simulink model "TestCellBalance"  (R2022b)
settings: Solver=VariableStepAuto  StartTime=0.0  StopTime=100  RelTol=1e-3
undefined symbols (not defined in the file): Ion, Lithium
libraries: spsSeriesRLCBranchLib x6, spsBatteryLib x4, spsVariableCapacitorLib x4, spsMosfetLib x4, spspowerguiLib x1
settings Model: Creator=49151  LastModifiedBy=49151
settings SolverCC: ZeroCrossAlgorithm=Adaptive
settings DebuggingCC: IgnoredZcDiagnostic=none

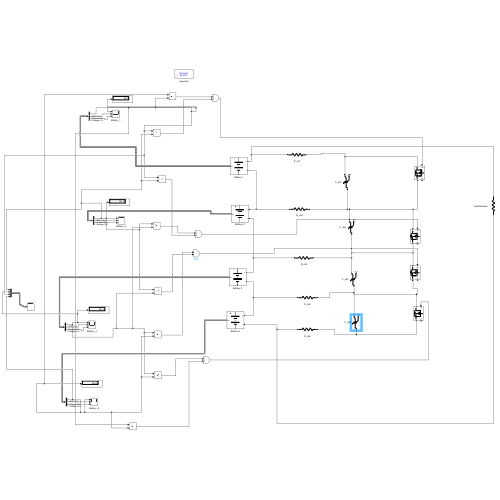
[thumbnail: Simulink's stored preview of the top-level diagram]
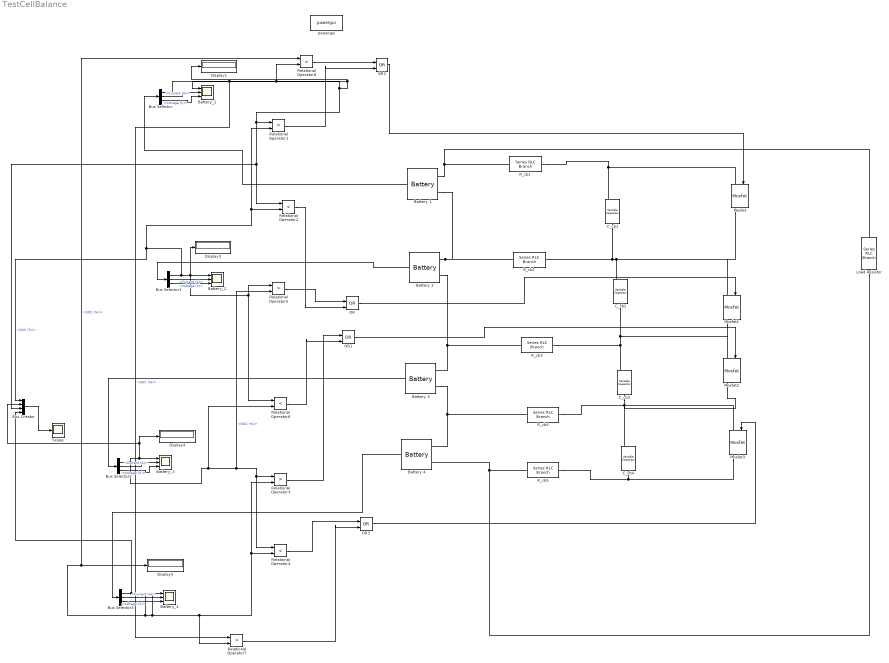
== system TestCellBalance ==
  Battery 1 : spsBatteryLib/Battery  BatType=Lithium-Ion  ShowTempParam=off  ThermalPreset=no  ShowAgeParam=off  NomV=3.7  NomQ=2.6  SOC=97  Batt_Tr=30  PresetModel=on  MaxQ=2.6  MinV=2.775  FullV=4.3068  Dis_rate=1.1304  R=0.014231  Normal_OP=2.3513  expZone="[3.9974     0.12774]"  current=[6.5 13 32.5]  Units=Time  Tci=20  NomT=20  T2=-30  MaxQ2=4.8  FullV2=7.1  Normal_OP2=5.655  expZone2="[6.58           1]"  Rca=0.6  ti=2000  Dp=0  Neq0=0  Tsim=1e6  Ta1=25  Qeol=5.4*0.9  Reol=0.013333*1.2  Char_age=[2.3478, 3]  Dis_age=[2.3478, 10]  N1=1500  N2=10500  N3=1000  N4=1400  Ta2=45  N5=950
  Battery 2 : spsBatteryLib/Battery  BatType=Lithium-Ion  ShowTempParam=off  ThermalPreset=no  ShowAgeParam=off  NomV=3.7  NomQ=2.6  SOC=96  Batt_Tr=30  PresetModel=on  MaxQ=2.6  MinV=2.775  FullV=4.3068  Dis_rate=1.1304  R=0.014231  Normal_OP=2.3513  expZone="[3.9974     0.12774]"  current=[6.5 13 32.5]  Units=Time  Tci=20  NomT=20  T2=-30  MaxQ2=4.8  FullV2=7.1  Normal_OP2=5.655  expZone2="[6.58           1]"  Rca=0.6  ti=2000  Dp=0  Neq0=0  Tsim=1e6  Ta1=25  Qeol=5.4*0.9  Reol=0.013333*1.2  Char_age=[2.3478, 3]  Dis_age=[2.3478, 10]  N1=1500  N2=10500  N3=1000  N4=1400  Ta2=45  N5=950
  Battery 3 : spsBatteryLib/Battery  BatType=Lithium-Ion  ShowTempParam=off  ThermalPreset=no  ShowAgeParam=off  NomV=3.7  NomQ=2.6  SOC=94  Batt_Tr=30  PresetModel=on  MaxQ=2.6  MinV=2.775  FullV=4.3068  Dis_rate=1.1304  R=0.014231  Normal_OP=2.3513  expZone="[3.9974     0.12774]"  current=[6.5 13 32.5]  Units=Time  Tci=20  NomT=20  T2=-30  MaxQ2=4.8  FullV2=7.1  Normal_OP2=5.655  expZone2="[6.58           1]"  Rca=0.6  ti=2000  Dp=0  Neq0=0  Tsim=1e6  Ta1=25  Qeol=5.4*0.9  Reol=0.013333*1.2  Char_age=[2.3478, 3]  Dis_age=[2.3478, 10]  N1=1500  N2=10500  N3=1000  N4=1400  Ta2=45  N5=950
  Battery 4 : spsBatteryLib/Battery  BatType=Lithium-Ion  ShowTempParam=off  ThermalPreset=no  ShowAgeParam=off  NomV=3.7  NomQ=2.6  SOC=96  Batt_Tr=30  PresetModel=on  MaxQ=2.6  MinV=2.775  FullV=4.3068  Dis_rate=1.1304  R=0.014231  Normal_OP=2.3513  expZone="[3.9974     0.12774]"  current=[6.5 13 32.5]  Units=Time  Tci=20  NomT=20  T2=-30  MaxQ2=4.8  FullV2=7.1  Normal_OP2=5.655  expZone2="[6.58           1]"  Rca=0.6  ti=2000  Dp=0  Neq0=0  Tsim=1e6  Ta1=25  Qeol=5.4*0.9  Reol=0.013333*1.2  Char_age=[2.3478, 3]  Dis_age=[2.3478, 10]  N1=1500  N2=10500  N3=1000  N4=1400  Ta2=45  N5=950
  Battery_{1..4} (4 alike) : Scope  NumInputPorts=3
  Bus Creator : BusCreator  Inputs=4
  Bus Selector{,1..3} (4 alike) : BusSelector  OutputSignals=SOC (%),Current (A),Voltage (V)
  C_cb{1..4} (4 alike) : spsVariableCapacitorLib/Variable Capacitor  methode=Backward Euler  Cabsmin=1e-6  Initialize=off  vC0=0  C0=1e-6  iC0=0
      settings: LibrarySourceBlock=sps_lib/Passives/Variable Capacitor
  Display{1,3..5} (4 alike) : Display
  Load Resistor : spsSeriesRLCBranchLib/Series RLC Branch  LConnTagsString=__new0  RConnTagsString=__new0  BranchType=R  Resistance=2  Inductance=1e-3  SetiL0=off  InitialCurrent=0  Capacitance=1e-6  Setx0=off  InitialVoltage=0  Measurements=None
  Mosfet{,1..3} (4 alike) : spsMosfetLib/Mosfet  Ron=0.1  Lon=0  Rd=0.01  Vfd=0  IC=0  Rs=1e5  Cs=inf  Measurements=on
  OR{,1..3} (4 alike) : Logic  Operator=OR  IconShape=distinctive  AllPortsSameDT=off  OutDataTypeStr=boolean
  R_cb{1..5} (5 alike) : spsSeriesRLCBranchLib/Series RLC Branch  LConnTagsString=__new0  RConnTagsString=__new0  BranchType=R  Resistance=1  Inductance=1e-3  SetiL0=off  InitialCurrent=0  Capacitance=1e-6  Setx0=off  InitialVoltage=0  Measurements=None
  Relational Operator{1,3,5,7} (4 alike) : RelationalOperator  Operator=>  OutDataTypeStr=boolean  RndMeth=Simplest  InputSameDT=off
  Relational Operator{2,4,6,8} (4 alike) : RelationalOperator  Operator=<  OutDataTypeStr=boolean  RndMeth=Simplest  InputSameDT=off
  Scope : Scope
  powergui : spspowerguiLib/powergui  Priority=1  SimulationMode=Discrete  SampleTime=50e-6  frequency=60  Iterations=50  frequencyindice=0  Pbase=100e6  ErrMax=1e-4  UnitsV=kV  UnitsW=MW  buscounter=0  FunctionMessages=off  echomessages=off  EnableUseOfTLC=off  CurrentSourceSwitches=off  DisableSnubberDevices=off  DisableRonSwitches=off  DisableVfSwitches=off  DisplayEquations=off  AutomaticDiscreteSolvers=off  SolverType=Tustin/Backward Euler (TBE)  Interpol=off  ExternalGateDelay=off  methode=off  Ts=100  x0status=blocks  SPID=on  SwTol=0  HookPort=off  NonlinearTolerance=1e-4  nMaxIteration=100  ContinueOnMaxIteration=off  RestoreLinks=warning  ResistiveCurrentMeasurement=off  Frange=[0:2:500]  Ylog=off  Xlog=on  ShowGrid=off  save=off  variable=ZData  structure=0  ZoomFFT=off  StartTime=0.0  cycles=1  DisplayStyle=1  fundamental=60  FreqAxis=off  MaxFrequency=1000  frequencyindicesteady=1  RmsSteady=1  display=off
  wires:
  Bus Selector/1 -> Bus Creator/3, Relational Operator2/1, Relational Operator1/1, Display1/1, Relational Operator8/2, Relational Operator7/1, Battery_1/1  "<SOC (%)>"
  Battery 1/1 -> Bus Selector/1
  Bus Selector/3 -> Battery_1/3  "<Voltage (V)>"
  Bus Selector/2 -> Battery_1/2  "<Current (A)>"
  Battery 2/1 -> Bus Selector1/1
  Bus Selector1/1 -> Relational Operator1/2, Relational Operator2/2, Bus Creator/1, Display3/1, Relational Operator5/1, Relational Operator6/1, Battery_2/1  "<SOC (%)>"
  Bus Selector1/2 -> Battery_2/2  "<Current (A)>"
  Bus Selector1/3 -> Battery_2/3  "<Voltage (V)>"
  Relational Operator2/1 -> OR/2
  Bus Selector3/3 -> Battery_4/3  "<Voltage (V)>"
  Bus Selector2/1 -> Battery_3/1, Bus Creator/2, Display4/1, Relational Operator6/2, Relational Operator5/2, Relational Operator4/1, Relational Operator3/1  "<SOC (%)>"
  Bus Selector2/3 -> Battery_3/3  "<Voltage (V)>"
  Battery 4/1 -> Bus Selector3/1
  Bus Selector3/2 -> Battery_4/2  "<Current (A)>"
  Bus Selector2/2 -> Battery_3/2  "<Current (A)>"
  Battery 3/1 -> Bus Selector2/1
  Bus Selector3/1 -> Bus Creator/4, Relational Operator7/2, Relational Operator3/2, Relational Operator4/2, Battery_4/1, Relational Operator8/1, Display5/1  "<SOC (%)>"
  Bus Creator/1 -> Scope/1
  Relational Operator5/1 -> OR/1
  OR/1 -> Mosfet1/1
  OR1/1 -> Mosfet2/1
  Relational Operator3/1 -> OR1/1
  Relational Operator6/1 -> OR1/2
  Relational Operator8/1 -> OR2/1
  Relational Operator1/1 -> OR2/2
  OR2/1 -> Mosfet/1
  Relational Operator4/1 -> OR3/1
  Relational Operator7/1 -> OR3/2
  OR3/1 -> Mosfet3/1
  connections:
  Battery 1/LConn1 -- Load Resistor/LConn1 -- R_cb1/LConn1
  Battery 2/LConn1 -- R_cb2/LConn1 -- Battery 1/LConn2
  R_cb5/LConn1 -- Load Resistor/RConn1 -- Battery 4/LConn2
  C_cb1/LConn1 -- R_cb1/RConn1 -- Mosfet/LConn1
  R_cb2/RConn1 -- C_cb1/RConn1 -- Mosfet/RConn1 -- Mosfet1/LConn1 -- C_cb2/LConn1
  R_cb3/RConn1 -- Mosfet2/LConn1 -- Mosfet1/RConn1 -- C_cb2/RConn1 -- C_cb3/LConn1
  R_cb4/RConn1 -- Mosfet2/RConn1 -- Mosfet3/LConn1 -- C_cb3/RConn1 -- C_cb4/LConn1
  R_cb5/RConn1 -- Mosfet3/RConn1 -- C_cb4/RConn1
  Battery 2/LConn2 -- Battery 3/LConn1 -- R_cb3/LConn1
  Battery 3/LConn2 -- Battery 4/LConn1 -- R_cb4/LConn1
